simulink model "ErrorSpaceSim"  (R2020b)
settings: Solver=ode45  StartTime=0.0  StopTime=5  RelTol=1e-3
undefined symbols (not defined in the file or in its folder): daq, degs2rpm, drv, es, gbox, mech, mld, mot, rads2rpm, rpm2rads, sens
settings Model: Creator=Utente  LastModifiedBy=Utente

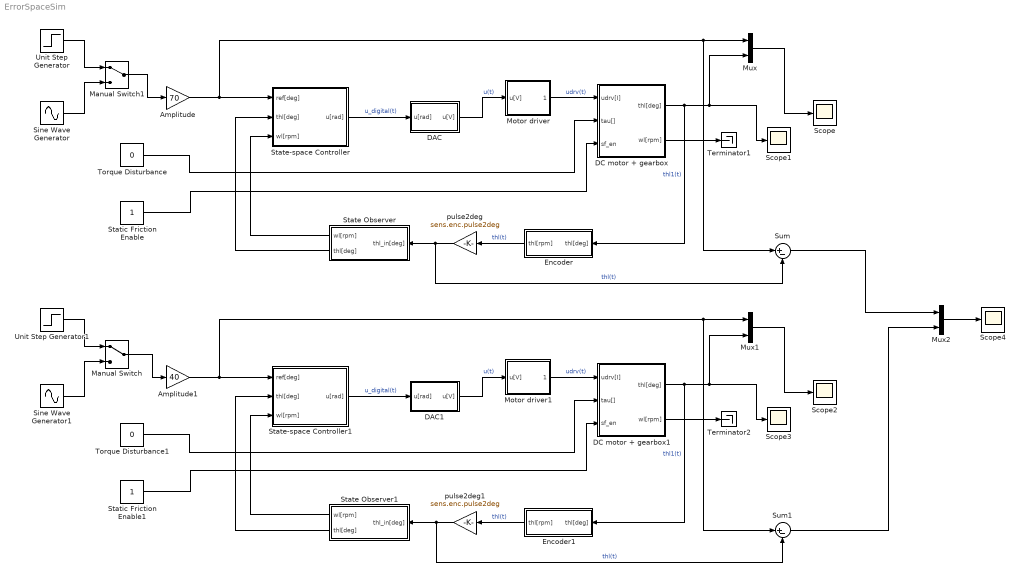
== system ErrorSpaceSim ==
  Amplitude : Gain  Gain=70
  Amplitude1 : Gain  Gain=40
  DAC : Subsystem
  DAC1 : Subsystem
  DC motor + gearbox : Subsystem
  DC motor + gearbox1 : Subsystem
  Encoder : Subsystem
  Encoder1 : Subsystem
  Manual Switch : ManualSwitch
  Manual Switch1 : ManualSwitch
  Motor driver : Subsystem
  Motor driver1 : Subsystem
  Mux : Mux  Inputs=2
  Mux1 : Mux  Inputs=2
  Mux2 : Mux  Inputs=2
  Scope{,1..4} (5 alike) : Scope
  Sine Wave Generator : Sin  Frequency=es.controller1.w0
  Sine Wave Generator1 : Sin  Frequency=2*pi/0.1
  State Observer : Subsystem
  State Observer1 : Subsystem
  State-space Controller : Subsystem
  State-space Controller1 : Subsystem
  Static Friction Enable : Constant
  Static Friction Enable1 : Constant
  Sum : Sum  Inputs=|+-
  Sum1 : Sum  Inputs=|+-
  Terminator1 : Terminator
  Terminator2 : Terminator
  Torque Disturbance : Constant  Value=0
  Torque Disturbance1 : Constant  Value=0
  Unit Step Generator : Step  Time=0  SampleTime=0
  Unit Step Generator1 : Step  Time=0  SampleTime=0
  pulse2deg : Gain  Gain=sens.enc.pulse2deg
  pulse2deg1 : Gain  Gain=sens.enc.pulse2deg
  wires:
  Motor driver/1(udrv[I]) -> DC motor + gearbox/1(udrv[I])  "udrv(t)"
  DAC/1(u[V]) -> Motor driver/1(u[V])  "u(t)"
  DC motor + gearbox/1(thl[deg]) -> Mux/2, Scope1/1, Encoder/1(thl[deg])  "thl1(t)"
  Encoder/1(thl[rpm]) -> pulse2deg/1  "thl(t)"
  State Observer/2(thl[deg]) -> State-space Controller/2(thl[deg])
  State-space Controller/1(u[rad]) -> DAC/1(u[rad])  "u_digital(t)"
  pulse2deg/1 -> Sum/2, State Observer/1(thl_in[deg])  "thl(t)"
  DC motor + gearbox/2(wl[rpm]) -> Terminator1/1
  State Observer/1(wl[rpm]) -> State-space Controller/3(wl[rpm])
  Amplitude/1 -> Sum/1, Mux/1, State-space Controller/1(ref[deg])
  Static Friction Enable/1 -> DC motor + gearbox/3(sf_en)
  Torque Disturbance/1 -> DC motor + gearbox/2(tau[])
  Mux/1 -> Scope/1
  Amplitude1/1 -> Sum1/1, Mux1/1, State-space Controller1/1(ref[deg])
  Mux1/1 -> Scope2/1
  State Observer1/1(wl[rpm]) -> State-space Controller1/3(wl[rpm])
  DC motor + gearbox1/1(thl[deg]) -> Mux1/2, Scope3/1, Encoder1/1(thl[deg])  "thl1(t)"
  DAC1/1(u[V]) -> Motor driver1/1(u[V])  "u(t)"
  Torque Disturbance1/1 -> DC motor + gearbox1/2(tau[])
  DC motor + gearbox1/2(wl[rpm]) -> Terminator2/1
  pulse2deg1/1 -> Sum1/2, State Observer1/1(thl_in[deg])  "thl(t)"
  State Observer1/2(thl[deg]) -> State-space Controller1/2(thl[deg])
  State-space Controller1/1(u[rad]) -> DAC1/1(u[rad])  "u_digital(t)"
  Static Friction Enable1/1 -> DC motor + gearbox1/3(sf_en)
  Motor driver1/1(udrv[I]) -> DC motor + gearbox1/1(udrv[I])  "udrv(t)"
  Encoder1/1(thl[rpm]) -> pulse2deg1/1  "thl(t)"
  Sum/1 -> Mux2/1
  Sum1/1 -> Mux2/2
  Mux2/1 -> Scope4/1
  Manual Switch/1 -> Amplitude1/1
  Unit Step Generator1/1 -> Manual Switch/1
  Sine Wave Generator1/1 -> Manual Switch/2
  Unit Step Generator/1 -> Manual Switch1/1
  Sine Wave Generator/1 -> Manual Switch1/2
  Manual Switch1/1 -> Amplitude/1

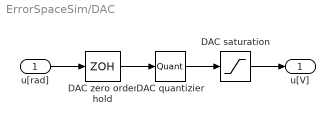
== system ErrorSpaceSim/DAC ==
  u[rad] : Inport
  DAC quantizier : Quantizer  QuantizationInterval=daq.dac.q
  DAC saturation : Saturate  UpperLimit=daq.dac.vdd  LowerLimit=daq.dac.vss
  DAC zero order hold : ZeroOrderHold  SampleTime=daq.dac.T_s
  u[V] : Outport
  wires:
  DAC quantizier/1 -> DAC saturation/1
  DAC zero order hold/1 -> DAC quantizier/1
  DAC saturation/1 -> u[V]/1
  u[rad]/1 -> DAC zero order hold/1

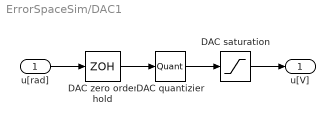
== system ErrorSpaceSim/DAC1 ==
  u[rad] : Inport
  DAC quantizier : Quantizer  QuantizationInterval=daq.dac.q
  DAC saturation : Saturate  UpperLimit=daq.dac.vdd  LowerLimit=daq.dac.vss
  DAC zero order hold : ZeroOrderHold  SampleTime=daq.dac.T_s
  u[V] : Outport
  wires:
  DAC quantizier/1 -> DAC saturation/1
  DAC zero order hold/1 -> DAC quantizier/1
  DAC saturation/1 -> u[V]/1
  u[rad]/1 -> DAC zero order hold/1

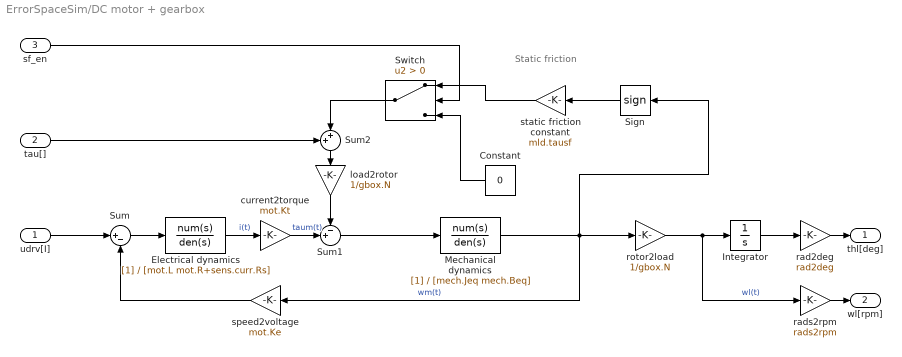
== system ErrorSpaceSim/DC motor + gearbox ==
  note: Static friction
  udrv[I] : Inport  Unit=V
  tau[] : Inport  Port=2  Unit=V
  sf_en : Inport  Port=3  Unit=V
  Constant : Constant  Value=0
  Electrical dynamics : TransferFcn  Denominator=[mot.L mot.R+sens.curr.Rs]
  Integrator : Integrator
  Mechanical dynamics : TransferFcn  Denominator=[mech.Jeq mech.Beq]
  Sign : Signum  ZeroCross=off
  Sum : Sum  Inputs=|+-
  Sum1 : Sum  Inputs=-+|
  Sum2 : Sum  Inputs=++|
  Switch : Switch  Criteria=u2 > Threshold
  current2torque : Gain  Gain=mot.Kt
  load2rotor : Gain  Gain=1/gbox.N
  rad2deg : Gain  Gain=rad2deg
  rads2rpm : Gain  Gain=rads2rpm
  rotor2load : Gain  Gain=1/gbox.N
  speed2voltage : Gain  Gain=mot.Ke
  static friction constant : Gain  Gain=mld.tausf
  thl[deg] : Outport  Unit=deg
  wl[rpm] : Outport  Port=2  Unit=rpm
  wires:
  load2rotor/1 -> Sum1/1
  Mechanical dynamics/1 -> Sign/1, rotor2load/1, speed2voltage/1  "wm(t)"
  Sign/1 -> static friction constant/1
  current2torque/1 -> Sum1/2  "taum(t)"
  Sum1/1 -> Mechanical dynamics/1
  speed2voltage/1 -> Sum/2
  rotor2load/1 -> rads2rpm/1, Integrator/1  "wl(t)"
  Electrical dynamics/1 -> current2torque/1  "i(t)"
  Integrator/1 -> rad2deg/1
  Sum/1 -> Electrical dynamics/1
  rads2rpm/1 -> wl[rpm]/1
  rad2deg/1 -> thl[deg]/1
  udrv[I]/1 -> Sum/1
  Sum2/1 -> load2rotor/1
  tau[]/1 -> Sum2/1
  Switch/1 -> Sum2/2
  static friction constant/1 -> Switch/1
  Constant/1 -> Switch/3
  sf_en/1 -> Switch/2

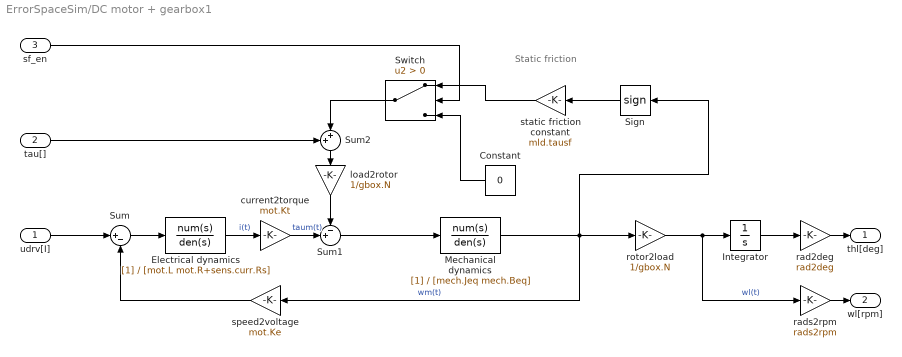
== system ErrorSpaceSim/DC motor + gearbox1 ==
  note: Static friction
  udrv[I] : Inport  Unit=V
  tau[] : Inport  Port=2  Unit=V
  sf_en : Inport  Port=3  Unit=V
  Constant : Constant  Value=0
  Electrical dynamics : TransferFcn  Denominator=[mot.L mot.R+sens.curr.Rs]
  Integrator : Integrator
  Mechanical dynamics : TransferFcn  Denominator=[mech.Jeq mech.Beq]
  Sign : Signum  ZeroCross=off
  Sum : Sum  Inputs=|+-
  Sum1 : Sum  Inputs=-+|
  Sum2 : Sum  Inputs=++|
  Switch : Switch  Criteria=u2 > Threshold
  current2torque : Gain  Gain=mot.Kt
  load2rotor : Gain  Gain=1/gbox.N
  rad2deg : Gain  Gain=rad2deg
  rads2rpm : Gain  Gain=rads2rpm
  rotor2load : Gain  Gain=1/gbox.N
  speed2voltage : Gain  Gain=mot.Ke
  static friction constant : Gain  Gain=mld.tausf
  thl[deg] : Outport  Unit=deg
  wl[rpm] : Outport  Port=2  Unit=rpm
  wires:
  load2rotor/1 -> Sum1/1
  Mechanical dynamics/1 -> Sign/1, rotor2load/1, speed2voltage/1  "wm(t)"
  Sign/1 -> static friction constant/1
  current2torque/1 -> Sum1/2  "taum(t)"
  Sum1/1 -> Mechanical dynamics/1
  speed2voltage/1 -> Sum/2
  rotor2load/1 -> rads2rpm/1, Integrator/1  "wl(t)"
  Electrical dynamics/1 -> current2torque/1  "i(t)"
  Integrator/1 -> rad2deg/1
  Sum/1 -> Electrical dynamics/1
  rads2rpm/1 -> wl[rpm]/1
  rad2deg/1 -> thl[deg]/1
  udrv[I]/1 -> Sum/1
  Sum2/1 -> load2rotor/1
  tau[]/1 -> Sum2/1
  Switch/1 -> Sum2/2
  static friction constant/1 -> Switch/1
  Constant/1 -> Switch/3
  sf_en/1 -> Switch/2

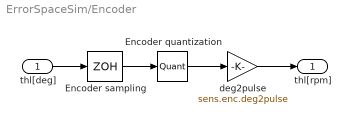
== system ErrorSpaceSim/Encoder ==
  thl[deg] : Inport
  Encoder quantization : Quantizer  QuantizationInterval=sens.enc.q
  Encoder sampling : ZeroOrderHold  SampleTime=sens.enc.T_s
  deg2pulse : Gain  Gain=sens.enc.deg2pulse
  thl[rpm] : Outport
  wires:
  Encoder quantization/1 -> deg2pulse/1
  deg2pulse/1 -> thl[rpm]/1
  Encoder sampling/1 -> Encoder quantization/1
  thl[deg]/1 -> Encoder sampling/1

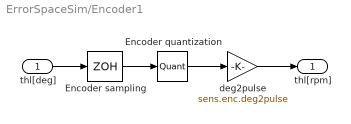
== system ErrorSpaceSim/Encoder1 ==
  thl[deg] : Inport
  Encoder quantization : Quantizer  QuantizationInterval=sens.enc.q
  Encoder sampling : ZeroOrderHold  SampleTime=sens.enc.T_s
  deg2pulse : Gain  Gain=sens.enc.deg2pulse
  thl[rpm] : Outport
  wires:
  Encoder quantization/1 -> deg2pulse/1
  deg2pulse/1 -> thl[rpm]/1
  Encoder sampling/1 -> Encoder quantization/1
  thl[deg]/1 -> Encoder sampling/1

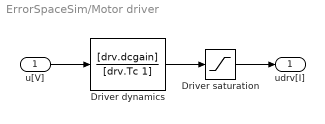
== system ErrorSpaceSim/Motor driver ==
  u[V] : Inport
  Driver dynamics : TransferFcn  Numerator=[drv.dcgain]  Denominator=[drv.Tc 1]
  Driver saturation : Saturate  UpperLimit=drv.vp  LowerLimit=drv.vm
  udrv[I] : Outport
  wires:
  Driver saturation/1 -> udrv[I]/1
  Driver dynamics/1 -> Driver saturation/1
  u[V]/1 -> Driver dynamics/1

== system ErrorSpaceSim/Motor driver1 ==
  u[V] : Inport
  Driver dynamics : TransferFcn  Numerator=[drv.dcgain]  Denominator=[drv.Tc 1]
  Driver saturation : Saturate  UpperLimit=drv.vp  LowerLimit=drv.vm
  udrv[I] : Outport
  wires:
  Driver saturation/1 -> udrv[I]/1
  Driver dynamics/1 -> Driver saturation/1
  u[V]/1 -> Driver dynamics/1

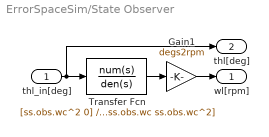
== system ErrorSpaceSim/State Observer ==
  thl_in[deg] : Inport
  Gain1 : Gain  Gain=degs2rpm
  Transfer Fcn : TransferFcn  Numerator=[ss.obs.wc^2 0]  Denominator=[1 2*ss.obs.delta*ss.obs.wc ss.obs.wc^2]
  wl[rpm] : Outport
  thl[deg] : Outport  Port=2
  wires:
  Transfer Fcn/1 -> Gain1/1
  thl_in[deg]/1 -> thl[deg]/1, Transfer Fcn/1
  Gain1/1 -> wl[rpm]/1

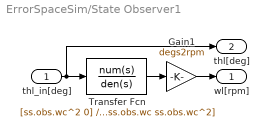
== system ErrorSpaceSim/State Observer1 ==
  thl_in[deg] : Inport
  Gain1 : Gain  Gain=degs2rpm
  Transfer Fcn : TransferFcn  Numerator=[ss.obs.wc^2 0]  Denominator=[1 2*ss.obs.delta*ss.obs.wc ss.obs.wc^2]
  wl[rpm] : Outport
  thl[deg] : Outport  Port=2
  wires:
  Transfer Fcn/1 -> Gain1/1
  thl_in[deg]/1 -> thl[deg]/1, Transfer Fcn/1
  Gain1/1 -> wl[rpm]/1

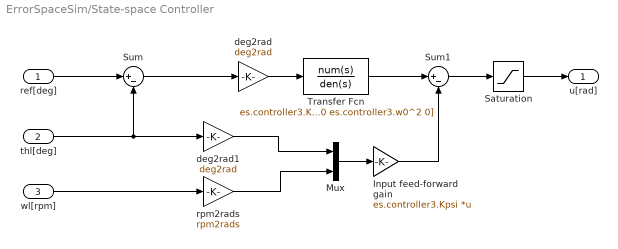
== system ErrorSpaceSim/State-space Controller ==
  ref[deg] : Inport
  thl[deg] : Inport  Port=2
  wl[rpm] : Inport  Port=3
  Input feed-forward gain : Gain  Gain=es.controller3.Kpsi  Multiplication=Matrix(K*u)
  Mux : Mux  Inputs=2
  Saturation : Saturate  UpperLimit=daq.dac.vdd  LowerLimit=daq.dac.vss
  Sum : Sum  Inputs=|+-
  Sum1 : Sum  Inputs=|+-
  Transfer Fcn : TransferFcn  Numerator=es.controller3.Kz  Denominator=[1 0 es.controller3.w0^2 0]
  deg2rad : Gain  Gain=deg2rad
  deg2rad1 : Gain  Gain=deg2rad
  rpm2rads : Gain  Gain=rpm2rads
  u[rad] : Outport
  wires:
  rpm2rads/1 -> Mux/2
  deg2rad1/1 -> Mux/1
  Saturation/1 -> u[rad]/1
  wl[rpm]/1 -> rpm2rads/1
  thl[deg]/1 -> Sum/2, deg2rad1/1
  deg2rad/1 -> Transfer Fcn/1
  Transfer Fcn/1 -> Sum1/1
  Input feed-forward gain/1 -> Sum1/2
  Mux/1 -> Input feed-forward gain/1
  Sum1/1 -> Saturation/1
  Sum/1 -> deg2rad/1
  ref[deg]/1 -> Sum/1

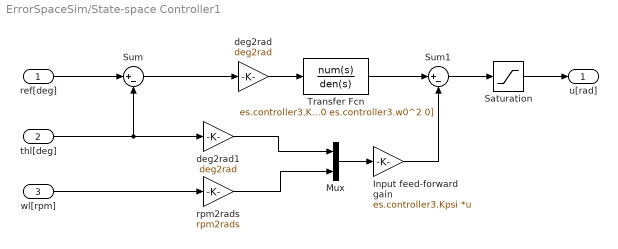
== system ErrorSpaceSim/State-space Controller1 ==
  ref[deg] : Inport
  thl[deg] : Inport  Port=2
  wl[rpm] : Inport  Port=3
  Input feed-forward gain : Gain  Gain=es.controller3.Kpsi  Multiplication=Matrix(K*u)
  Mux : Mux  Inputs=2
  Saturation : Saturate  UpperLimit=daq.dac.vdd  LowerLimit=daq.dac.vss
  Sum : Sum  Inputs=|+-
  Sum1 : Sum  Inputs=|+-
  Transfer Fcn : TransferFcn  Numerator=es.controller3.Kz  Denominator=[1 0 es.controller3.w0^2 0]
  deg2rad : Gain  Gain=deg2rad
  deg2rad1 : Gain  Gain=deg2rad
  rpm2rads : Gain  Gain=rpm2rads
  u[rad] : Outport
  wires:
  rpm2rads/1 -> Mux/2
  deg2rad1/1 -> Mux/1
  Saturation/1 -> u[rad]/1
  wl[rpm]/1 -> rpm2rads/1
  thl[deg]/1 -> Sum/2, deg2rad1/1
  deg2rad/1 -> Transfer Fcn/1
  Transfer Fcn/1 -> Sum1/1
  Input feed-forward gain/1 -> Sum1/2
  Mux/1 -> Input feed-forward gain/1
  Sum1/1 -> Saturation/1
  Sum/1 -> deg2rad/1
  ref[deg]/1 -> Sum/1
